simulink model "Likitha_Version_10"  (R2025b)
settings: Solver=VariableStepAuto  StartTime=0.0  StopTime=0.3  RelTol=1e-3
undefined symbols (not defined in the file or in its folder): Ion, Lithium
libraries: spsBatteryLib x50, spsSeriesRLCBranchLib x15, spsCurrentMeasurementLib x10, spsVoltageMeasurementLib x10, spsIdealSwitchLib x9, spsMosfetLib x7, slpidlib x4, spsPWMGeneratorDCDCLib x2, spspowerguiLib x2, spsACVoltageSourceLib x1, eeHysteresisControl x1, spsDCMachineLib x1
(part 5 of 5)

== matlab function Likitha_Version_10/Subsystem6/MATLAB Function ==
  settings: updateMethod=DISCRETE
  data: sim_params input double size=[1 22]; V_dif output double size=1; hw_params input double size=[1 22]; timestamp input double size=1; sim_algo input double size=1; hw_algo input double size=1; reset input double size=1; I_dif output double size=1; P_dif output double size=1; SOC_dif output double size=1; SCH_dif output double size=1; mse_V output double size=1; mse_I output double size=1; mse_SOC output double size=1; mse_SCH output double size=1; max_cell_imbalance_sim output double size=1; max_cell_imbalance_hv output double size=1; charging_efficiency output double size=1; discharging_efficiency output double size=1; coulombic_efficiency output double size=1; slg2_sim output double size=1; algo_hv output double size=1; log_data output double size=[1 66]
function [V_dif, I_dif, P_dif, SOC_dif, SCH_dif, ...
          mse_V, mse_I, mse_SOC, mse_SCH, ...
          max_cell_imbalance_sim, max_cell_imbalance_hv, ...
          charging_efficiency, discharging_efficiency, coulombic_efficiency, ...
          slg2_sim, algo_hv, log_data] = ...
    CompareModules_Final(sim_params, hw_params, timestamp, sim_algo, hw_algo, reset)

% Comparison Block – fixed‑size persistent arrays, code‑generation ready
% Inputs:
%   sim_params : [1x22] vector from simulation branch
%   hw_params  : [1x22] vector from hardware branch
%   timestamp  : current simulation time (scalar)
%   sim_algo   : algorithm code for simulation (scalar)
%   hw_algo    : algorithm code for hardware (scalar)
%   reset      : set to 1 to reset accumulated errors (scalar)
%
% Outputs (17 total):
%   V_dif, I_dif, P_dif, SOC_dif, SCH_dif : instantaneous differences
%   mse_V, mse_I, mse_SOC, mse_SCH        : running RMSE
%   max_cell_imbalance_sim, max_cell_imbalance_hv : cell voltage spreads
%   charging_efficiency, discharging_efficiency, coulombic_efficiency
%   slg2_sim, algo_hv                      : algorithm codes
%   log_data                                : [1x66] vector for CSV logging

% -------------------------------------------------------------------------
% Parameter index mapping (1‑based) – MUST match your upstream blocks
% 1:SOC, 2:SOH, 3:SOP, 4:DOD, 5:ROH, 6:RUL, 7:CycleCount,
% 8:V_avg, 9:I_avg, 10:P_avg, 11:stress_idx, 12:aging_rate_frac, 13:energy_kWh,
% 14:degrad_idx, 15:T_idx, 16:health_idx, 17:I_peak, 18:V_min, 19:T_max,
% 20:Ah_charge_total, 21:Ah_discharge_total, 22:overtime_sec
% -------------------------------------------------------------------------

% Extract simulation parameters
SOC_sim   = sim_params(1);
SOH_sim   = sim_params(2);
RUL_sim   = sim_params(6);
Cycle_sim = sim_params(7);
V_sim     = sim_params(8);
I_sim     = sim_params(9);
P_sim     = sim_params(10);
stress_sim = sim_params(11);
health_sim = sim_params(16);
V_min_sim  = sim_params(18);
V_max_sim  = sim_params(17);   % using I_peak as proxy for max voltage
T_sim      = sim_params(19);   % T_max as temperature proxy
energy_sim = sim_params(13);
charge_sim = sim_params(20) + sim_params(21); % total Ah throughput

% Extract hardware parameters (same indices)
SOC_hw   = hw_params(1);
SOH_hw   = hw_params(2);
RUL_hw   = hw_params(6);
Cycle_hw = hw_params(7);
V_hw     = hw_params(8);
I_hw     = hw_params(9);
P_hw     = hw_params(10);
stress_hw = hw_params(11);
health_hw = hw_params(16);
V_min_hw  = hw_params(18);
V_max_hw  = hw_params(17);
T_hw      = hw_params(19);
energy_hw = hw_params(13);
charge_hw = hw_params(20) + hw_params(21);

% Compute instantaneous differences
V_dif   = V_sim - V_hw;
I_dif   = I_sim - I_hw;
P_dif   = P_sim - P_hw;
SOC_dif = SOC_sim - SOC_hw;
SCH_dif = SOH_sim - SOH_hw;
T_dif   = T_sim - T_hw;          % for logging only
Cycle_dif = Cycle_sim - Cycle_hw;
RUL_dif   = RUL_sim - RUL_hw;
health_dif = health_sim - health_hw;
stress_dif = stress_sim - stress_hw;

% -------------------------------------------------------------------------
% Persistent variables for RMSE (fixed‑size circular buffer)
persistent err_V err_I err_SOC err_SOH err_idx max_errors
persistent cum_energy_sim cum_energy_hw cum_charge_sim cum_charge_hw

% Initialize on first call
if isempty(err_V)
    max_errors = 10000;                        % store up to 10000 samples
    err_V = zeros(1, max_errors);
    err_I = zeros(1, max_errors);
    err_SOC = zeros(1, max_errors);
    err_SOH = zeros(1, max_errors);
    err_idx = 0;
    cum_energy_sim = 0;
    cum_energy_hw  = 0;
    cum_charge_sim = 0;
    cum_charge_hw  = 0;
elseif reset
    % Reinitialize when reset is triggered
    err_V(:) = 0;
    err_I(:) = 0;
    err_SOC(:) = 0;
    err_SOH(:) = 0;
    err_idx = 0;
    cum_energy_sim = 0;
    cum_energy_hw  = 0;
    cum_charge_sim = 0;
    cum_charge_hw  = 0;
end

% Update cumulative values with latest parameters (these are just copies)
cum_energy_sim = energy_sim;
cum_energy_hw  = energy_hw;
cum_charge_sim = charge_sim;
cum_charge_hw  = charge_hw;

% Store errors only when timestamp advances (and not reset)
if timestamp > 0 && ~reset
    err_idx = err_idx + 1;
    if err_idx > max_errors
        % Circular buffer: discard oldest, keep most recent
        err_V(1:end-1) = err_V(2:end);
        err_I(1:end-1) = err_I(2:end);
        err_SOC(1:end-1) = err_SOC(2:end);
        err_SOH(1:end-1) = err_SOH(2:end);
        err_idx = max_errors;
    end
    err_V(err_idx) = V_dif;
    err_I(err_idx) = I_dif;
    err_SOC(err_idx) = SOC_dif;
    err_SOH(err_idx) = SCH_dif;
end

% Compute RMSE from all stored errors
if err_idx > 0
    mse_V   = sqrt(mean(err_V(1:err_idx).^2));
    mse_I   = sqrt(mean(err_I(1:err_idx).^2));
    mse_SOC = sqrt(mean(err_SOC(1:err_idx).^2));
    mse_SCH = sqrt(mean(err_SOH(1:err_idx).^2));
else
    mse_V = 0; mse_I = 0; mse_SOC = 0; mse_SCH = 0;
end

% Cell imbalance (using min and max as proxy)
max_cell_imbalance_sim = V_max_sim - V_min_sim;
max_cell_imbalance_hv  = V_max_hw  - V_min_hw;

% Efficiencies (prevent division by zero)
if cum_energy_hw > 0
    charging_efficiency = cum_energy_sim / cum_energy_hw;
else
    charging_efficiency = 1;
end
if cum_charge_hw > 0
    coulombic_efficiency = cum_charge_sim / cum_charge_hw;
else
    coulombic_efficiency = 1;
end
discharging_efficiency = charging_efficiency; % simplified

% Algorithm codes
slg2_sim = sim_algo;
algo_hv  = hw_algo;

% -------------------------------------------------------------------------
% Build log_data vector – fixed length 1x66
% Order:
%   1 timestamp
%   2-23 sim_params (22)
%   24-45 hw_params (22)
%   46 V_dif, 47 I_dif, 48 P_dif, 49 SOC_dif, 50 SCH_dif,
%   51 T_dif, 52 Cycle_dif, 53 RUL_dif, 54 health_dif, 55 stress_dif
%   56 mse_V, 57 mse_I, 58 mse_SOC, 59 mse_SCH
%   60 max_cell_imbalance_sim, 61 max_cell_imbalance_hv
%   62 charging_efficiency, 63 discharging_efficiency, 64 coulombic_efficiency
%   65 sim_algo, 66 hw_algo
% -------------------------------------------------------------------------
log_data = [timestamp, ...
            sim_params, ...
            hw_params, ...
            V_dif, I_dif, P_dif, SOC_dif, SCH_dif, T_dif, Cycle_dif, RUL_dif, health_dif, stress_dif, ...
            mse_V, mse_I, mse_SOC, mse_SCH, ...
            max_cell_imbalance_sim, max_cell_imbalance_hv, ...
            charging_efficiency, discharging_efficiency, coulombic_efficiency, ...
            sim_algo, hw_algo];

end

== matlab function Likitha_Version_10/Subsystem8/MATLAB Function ==
  data: in1 input; out1 output; in2 input; in3 input; in4 input; in5 input; in6 input; in7 input; in8 input; in9 input; in10 input; in11 input; in12 input; in13 input; in14 input; in15 input; in16 input; in17 input; in18 input; in19 input; in20 input; in21 input; in22 input; in23 input; in24 input; in25 input; in26 input; in27 input; in28 input; in29 input; in30 input; in31 input; in32 input; out2 output; out3 output; out4 output; out5 output; out6 output; out7 output; out8 output; out9 output; out10 output; out11 output; out12 output; out13 output; out14 output; out15 output; out16 output; out17 output; out18 output; out19 output; out20 output; out21 output; out22 output; out23 output; out24 output; out25 output; out26 output; out27 output; out28 output; out29 output; out30 output; out31 output; out32 output
function [out1, out2, out3, out4, out5, out6, out7, out8, ...
          out9, out10, out11, out12, out13, out14, out15, out16, ...
          out17, out18, out19, out20, out21, out22, out23, out24, ...
          out25, out26, out27, out28, out29, out30, out31, out32] = ...
    FineTune32(in1, in2, in3, in4, in5, in6, in7, in8, ...
               in9, in10, in11, in12, in13, in14, in15, in16, ...
               in17, in18, in19, in20, in21, in22, in23, in24, ...
               in25, in26, in27, in28, in29, in30, in31, in32)

% Fine‑Tune 32 Outputs – corrects zeros, computes missing RMSE, adds novelty
% All persistent variables are fixed‑size arrays (code‑generation friendly)

% -------------------------------------------------------------------------
% Map inputs to meaningful names
V_sim        = in1;   I_sim        = in2;   SOC_sim      = in3;   SOH_sim      = in4;
T_sim        = in5;   RUL_sim      = in6;   health_sim   = in7;   V_hw         = in8;
I_hw         = in9;   SOC_hw       = in10;  SOH_hw       = in11;  T_hw         = in12;
RUL_hw       = in13;  health_hw    = in14;  V_diff       = in15;  I_diff       = in16;
SOC_diff     = in17;  SOH_diff     = in18;  T_diff       = in19;  RUL_diff     = in20;
RMSE_V       = in21;  RMSE_I       = in22;  RMSE_SOC     = in23;  RMSE_SOH     = in24;
imbalance_sim= in25;  imbalance_hw = in26;  charging_eff = in27;  coulombic_eff= in28;
algo_sim     = in29;  algo_hw      = in30;  stress_sim   = in31;  stress_hw    = in32;

% -------------------------------------------------------------------------
% Persistent variables for RMSE calculation (fixed‑size circular buffer)
persistent err_V err_I err_SOC err_SOH err_idx max_errors
persistent initialized

% Initialize on first call
if isempty(initialized)
    max_errors = 1000;                     % store up to 1000 samples
    err_V = zeros(1, max_errors);
    err_I = zeros(1, max_errors);
    err_SOC = zeros(1, max_errors);
    err_SOH = zeros(1, max_errors);
    err_idx = 0;
    initialized = true;
end

% Update error history if differences are non‑zero
if abs(V_diff) > 1e-6 || abs(I_diff) > 1e-6 || abs(SOC_diff) > 1e-6 || abs(SOH_diff) > 1e-6
    err_idx = err_idx + 1;
    if err_idx > max_errors
        % Shift buffer: discard oldest, keep most recent
        err_V(1:end-1) = err_V(2:end);
        err_I(1:end-1) = err_I(2:end);
        err_SOC(1:end-1) = err_SOC(2:end);
        err_SOH(1:end-1) = err_SOH(2:end);
        err_idx = max_errors;
    end
    err_V(err_idx) = V_diff;
    err_I(err_idx) = I_diff;
    err_SOC(err_idx) = SOC_diff;
    err_SOH(err_idx) = SOH_diff;
end

% -------------------------------------------------------------------------
% Fine‑tune each output
% -------------------------------------------------------------------------

% 1. Simulation core – realistic bounds
V_sim    = max(0, min(500, V_sim));
I_sim    = max(-100, min(100, I_sim));
SOC_sim  = max(0, min(100, SOC_sim));
SOH_sim  = max(0, min(100, SOH_sim));
T_sim    = max(-20, min(80, T_sim));
RUL_sim  = max(0, RUL_sim);
health_sim = max(0, min(1, health_sim));

% 2. Hardware core
V_hw    = max(0, min(500, V_hw));
I_hw    = max(-100, min(100, I_hw));
SOC_hw  = max(0, min(100, SOC_hw));
SOH_hw  = max(0, min(100, SOH_hw));
T_hw    = max(-20, min(80, T_hw));
RUL_hw  = max(0, RUL_hw);
health_hw = max(0, min(1, health_hw));

% 3. Differences – recompute for consistency
V_diff   = V_sim - V_hw;
I_diff   = I_sim - I_hw;
SOC_diff = SOC_sim - SOC_hw;
SOH_diff = SOH_sim - SOH_hw;
T_diff   = T_sim - T_hw;
RUL_diff = RUL_sim - RUL_hw;

% 4. RMSE – if input is zero but we have history, compute it
if (RMSE_V == 0 || RMSE_I == 0 || RMSE_SOC == 0 || RMSE_SOH == 0) && err_idx > 0
    if RMSE_V == 0,   RMSE_V   = sqrt(mean(err_V(1:err_idx).^2));   end
    if RMSE_I == 0,   RMSE_I   = sqrt(mean(err_I(1:err_idx).^2));   end
    if RMSE_SOC == 0, RMSE_SOC = sqrt(mean(err_SOC(1:err_idx).^2)); end
    if RMSE_SOH == 0, RMSE_SOH = sqrt(mean(err_SOH(1:err_idx).^2)); end
end
RMSE_V   = max(0, RMSE_V);
RMSE_I   = max(0, RMSE_I);
RMSE_SOC = max(0, RMSE_SOC);
RMSE_SOH = max(0, RMSE_SOH);

% 5. Imbalance – ensure non‑negative
imbalance_sim = max(0, imbalance_sim);
imbalance_hw  = max(0, imbalance_hw);

% 6. Efficiencies – clamp between 0 and 2
charging_eff   = max(0, min(2, charging_eff));
coulombic_eff  = max(0, min(2, coulombic_eff));

% 7. Algorithm codes – keep as integers 1‑5
algo_sim = round(max(1, min(5, algo_sim)));
algo_hw  = round(max(1, min(5, algo_hw)));

% 8. Stress indices – clamp 0‑1
stress_sim = max(0, min(1, stress_sim));
stress_hw  = max(0, min(1, stress_hw));

% -------------------------------------------------------------------------
% Optional novelty: composite Digital Twin Health Score (example)
dt_health_score = 0.5 * (health_sim + health_hw) / 2 ...
                + 0.3 * (1 - tanh(RMSE_SOC / 5)) ...
                + 0.2 * (1 - tanh(abs(SOC_diff) / 10));
dt_health_score = max(0, min(1, dt_health_score));
% You could replace one output with this score, e.g., out32 = dt_health_score;

% -------------------------------------------------------------------------
% Assign outputs (same order as inputs)
out1  = V_sim;        out2  = I_sim;        out3  = SOC_sim;      out4  = SOH_sim;
out5  = T_sim;        out6  = RUL_sim;      out7  = health_sim;   out8  = V_hw;
out9  = I_hw;         out10 = SOC_hw;       out11 = SOH_hw;       out12 = T_hw;
out13 = RUL_hw;       out14 = health_hw;    out15 = V_diff;       out16 = I_diff;
out17 = SOC_diff;     out18 = SOH_diff;     out19 = T_diff;       out20 = RUL_diff;
out21 = RMSE_V;       out22 = RMSE_I;       out23 = RMSE_SOC;     out24 = RMSE_SOH;
out25 = imbalance_sim; out26 = imbalance_hw; out27 = charging_eff; out28 = coulombic_eff;
out29 = algo_sim;     out30 = algo_hw;      out31 = stress_sim;   out32 = stress_hw;

% (Optional: replace out32 with dt_health_score)
% out32 = dt_health_score;

end

== matlab function Likitha_Version_10/Controller/BMS ==
  settings: updateMethod=DISCRETE
  data: SOC input; C output; t input
function C = fcn_charge_discharge_time(SOC, t)
% C = 1 → Charge
% C = 0 → Discharge

%% USER SETTINGS
T_charge    = 100;   % Charge duration (sec)
T_discharge = 100;   % Discharge duration (sec)
MaxCycles   = 5;     % Number of cycles

%% Persistent variables
persistent last_value t_ref cycle mode
% mode: 1 = charge, 0 = discharge

if isempty(last_value)
    last_value = 1;      % Start with charging
    t_ref = t;
    cycle = 0;
    mode = 1;
end

%% Stop switching after max cycles
if cycle >= MaxCycles
    C = last_value;
    return;
end

%% Time-based switching
if mode == 1   % Charging
    if (t - t_ref) >= T_charge || SOC >= 80
        mode = 0;       % Switch to discharge
        t_ref = t;
    end
else           % Discharging
    if (t - t_ref) >= T_discharge || SOC <= 20
        mode = 1;       % Switch to charge
        t_ref = t;
        cycle = cycle + 1;  % Count full cycle
    end
end

%% Output
C = mode;
last_value = C;

end

== matlab function Likitha_Version_10/Subsystem11/Subsystem/MATLAB Function ==
  data: inputValue input; output output
function output = divideByFifty(inputValue)
% This function divides the input decimal value by 50

output = inputValue / 50;

end

== stateflow chart Likitha_Version_10/Charger/5SCCC ==
  state Initialize
    entry:
    signal=1;
    Iref=1*C;
  state fifth_stage
    entry:
    Iref=0.01*C;
  state end
    entry:
    signal=2;
  state back_to_charge
    entry:
    signal=1;
    Iref=0;
  state first_stage
    entry:
    Iref=0.32*C;
  state fourth_stage
    entry:
    Iref=0.057*C;
  state second_stage
    entry:
    Iref=0.1*C;
  state third_stage
    entry:
    Iref=0.1*C;
  back_to_charge -> (junction 27)
  (junction 27) -> end [order 2]
  (default) -> (junction 27)
  Initialize -> (junction 27) [order 2] : [sw==0]
  (junction 27) -> Initialize [order 1] : [sw==1]
  end -> back_to_charge : [sw==1]
  fifth_stage -> end [order 1] : [Vpeak<=Vb]
  first_stage -> Initialize [order 2] : [sw==0]
  fifth_stage -> fourth_stage [order 2] : [sw==0]
  Initialize -> first_stage [order 1] : [Vpeak<=Vb]
  fourth_stage -> fifth_stage [order 1] : [Vpeak<=Vb]
  fourth_stage -> third_stage [order 2] : [sw==0]
  second_stage -> first_stage [order 2] : [sw==0]
  first_stage -> second_stage [order 1] : [Vpeak<=Vb]
  third_stage -> fourth_stage [order 1] : [Vpeak<=Vb]
  second_stage -> third_stage [order 1] : [Vpeak<=Vb]
  third_stage -> second_stage [order 2] : [sw==0]
  data: Vpeak input; Vb input; Iref output; signal output; C input; sw input
